simulink model "sim_01_a_RightSide"  (R2022a)
settings: Solver=VariableStepAuto  StartTime=0.0  StopTime=25  RelTol=1e-3
settings Model: Creator=Eshmith  LastModifiedBy=Eshmith

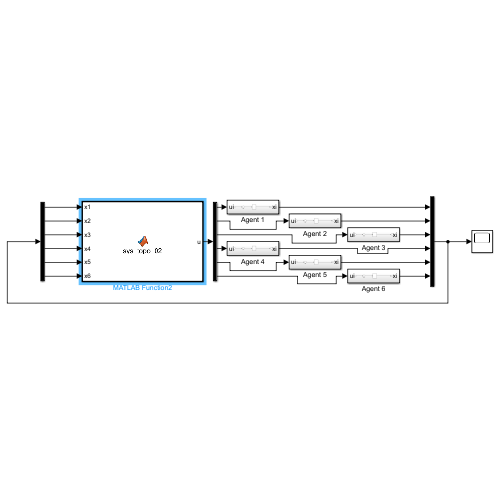
[thumbnail: Simulink's stored preview of the top-level diagram]
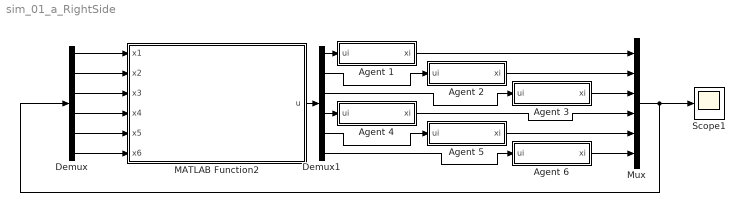
== system sim_01_a_RightSide ==
  Agent 1 : Subsystem
  Agent 2 : Subsystem
  Agent 3 : Subsystem
  Agent 4 : Subsystem
  Agent 5 : Subsystem
  Agent 6 : Subsystem
  Demux : Demux  Outputs=6
  Demux1 : Demux  Outputs=6
  MATLAB Function2 : MATLAB Function  TreatAsAtomicUnit=on
  Mux : Mux  Inputs=6
  Scope1 : Scope
  wires:
  Mux/1 -> Demux/1, Scope1/1
  Demux1/1 -> Agent 1/1(ui)
  MATLAB Function2/1(u) -> Demux1/1
  Agent 1/1(xi) -> Mux/1
  Agent 6/1(xi) -> Mux/6
  Agent 4/1(xi) -> Mux/4
  Demux1/3 -> Agent 3/1(ui)
  Demux/3 -> MATLAB Function2/3(x3)
  Demux1/2 -> Agent 2/1(ui)
  Agent 5/1(xi) -> Mux/5
  Demux/4 -> MATLAB Function2/4(x4)
  Demux/6 -> MATLAB Function2/6(x6)
  Demux1/4 -> Agent 4/1(ui)
  Demux1/6 -> Agent 6/1(ui)
  Demux/5 -> MATLAB Function2/5(x5)
  Agent 3/1(xi) -> Mux/3
  Demux/2 -> MATLAB Function2/2(x2)
  Demux/1 -> MATLAB Function2/1(x1)
  Demux1/5 -> Agent 5/1(ui)
  Agent 2/1(xi) -> Mux/2

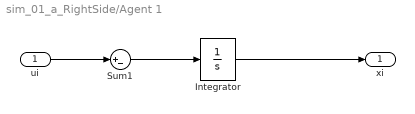
== system sim_01_a_RightSide/Agent 1 ==
  ui : Inport
  Integrator : Integrator  InitialCondition=10
  Sum1 : Sum  Inputs=|+-
  xi : Outport
  wires:
  Sum1/1 -> Integrator/1
  ui/1 -> Sum1/1
  Integrator/1 -> xi/1

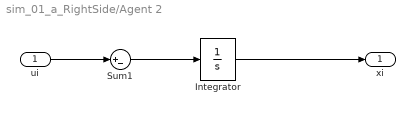
== system sim_01_a_RightSide/Agent 2 ==
  ui : Inport
  Integrator : Integrator  InitialCondition=1
  Sum1 : Sum  Inputs=|+-
  xi : Outport
  wires:
  Sum1/1 -> Integrator/1
  ui/1 -> Sum1/1
  Integrator/1 -> xi/1

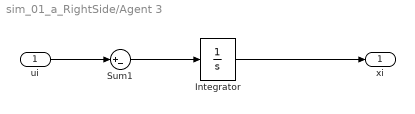
== system sim_01_a_RightSide/Agent 3 ==
  ui : Inport
  Integrator : Integrator  InitialCondition=2
  Sum1 : Sum  Inputs=|+-
  xi : Outport
  wires:
  Sum1/1 -> Integrator/1
  ui/1 -> Sum1/1
  Integrator/1 -> xi/1

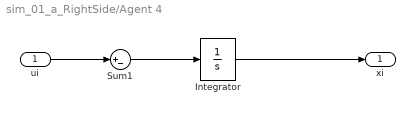
== system sim_01_a_RightSide/Agent 4 ==
  ui : Inport
  Integrator : Integrator  InitialCondition=3
  Sum1 : Sum  Inputs=|+-
  xi : Outport
  wires:
  Sum1/1 -> Integrator/1
  ui/1 -> Sum1/1
  Integrator/1 -> xi/1

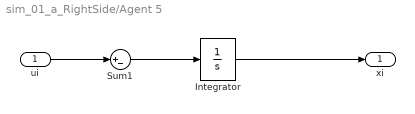
== system sim_01_a_RightSide/Agent 5 ==
  ui : Inport
  Integrator : Integrator  InitialCondition=4
  Sum1 : Sum  Inputs=|+-
  xi : Outport
  wires:
  Sum1/1 -> Integrator/1
  ui/1 -> Sum1/1
  Integrator/1 -> xi/1

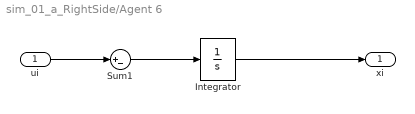
== system sim_01_a_RightSide/Agent 6 ==
  ui : Inport
  Integrator : Integrator  InitialCondition=5
  Sum1 : Sum  Inputs=|+-
  xi : Outport
  wires:
  Sum1/1 -> Integrator/1
  ui/1 -> Sum1/1
  Integrator/1 -> xi/1

== matlab function sim_01_a_RightSide/MATLAB Function2 ==
  data: x1 input; u output; x2 input; x3 input; x4 input; x5 input; x6 input
function u = sys_topo_02(x1, x2, x3, x4, x5, x6)

L = [+1  0  0  0  0 -1;
     -1 +1  0  0  0  0;
      0 -1 +1  0  0  0;
      0  0 -1 +1  0  0;
      0  0  0 -1 +1  0;
      0  0  0  0 -1 +1;
       ];

states = [x1, x2, x3, x4, x5, x6]';

u = -L*states;

end
